simulink model "controller_lon2"  (R2017b)
settings: Solver=VariableStepAuto  StartTime=0.0  StopTime=10  RelTol=1e-3
values from neighbouring files (symbols this model uses):
  CSim_theta = 1    [controller_lon_design.m]
  KF_theta = 0.000000    (= 0)    [controller_lon_design.m]    (also in lon_gain20190526.mat = -0.572510862227)
  KI_theta = 0.3    [controller_lon_design.m]    (also in lon_gain20190526.mat = 0.842649674918)
  KP_q = 1.7    [controller_lon_design.m]    (also in lon_gain20190526.mat = 1.88196418813)
  KP_q2 = 0.3    [controller_lon_design.m]    (also in lon_gain20190526.mat = 0.215046441763)
  KP_theta = 1.2    [controller_lon_design.m]    (also in lon_gain20190526.mat = 0.644469729819)
undefined symbols (not defined in the file or in its folder): Actuators, Linmod
settings Model: Creator=zht  LastModifiedBy=zht

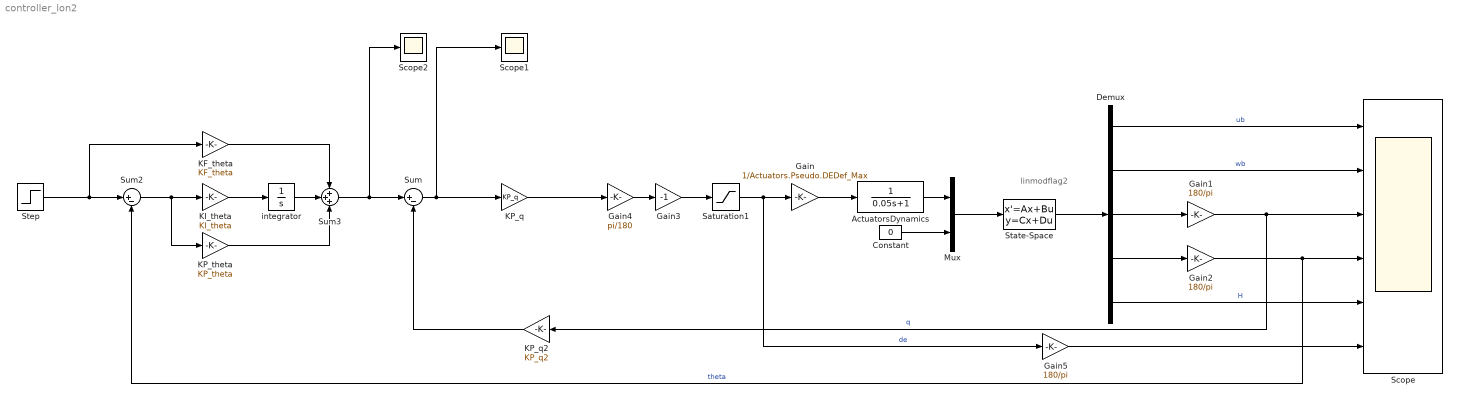
== system controller_lon2 ==
  note: linmodflag2
  ActuatorsDynamics : TransferFcn  Denominator=[0.05 1]
  Constant : Constant  Value=0
  Demux : Demux  Outputs=5
  Gain : Gain  Gain=1/Actuators.Pseudo.DEDef_Max
  Gain1 : Gain  Gain=180/pi
  Gain2 : Gain  Gain=180/pi
  Gain3 : Gain  Gain=-1
  Gain4 : Gain  Gain=pi/180
  Gain5 : Gain  Gain=180/pi
  KF_theta : Gain  Gain=KF_theta
  KI_theta : Gain  Gain=KI_theta
  KP_q : Gain  Gain=KP_q
  KP_q2 : Gain  Gain=KP_q2
  KP_theta : Gain  Gain=KP_theta
  Mux : Mux  Inputs=2
  Saturation1 : Saturate  UpperLimit=Actuators.Pseudo.DEDef_Max  LowerLimit=-Actuators.Pseudo.DEDef_Max
  Scope : Scope  NumInputPorts=6
  Scope1 : Scope
  Scope2 : Scope
  State-Space : StateSpace  A=Linmod.Lon_5.A  B=Linmod.Lon_5.B  C=Linmod.Lon_5.C  D=Linmod.Lon_5.D  InitialCondition=0  ContinuousStateAttributes={'ub','wb','q','theta','H'}
  Step : Step  Time=0  After=CSim_theta  SampleTime=0
  Sum : Sum  Inputs=|+-
  Sum2 : Sum  Inputs=|+-
  Sum3 : Sum  Inputs=+++
  integrator : Integrator
  wires:
  Mux/1 -> State-Space/1
  Constant/1 -> Mux/2
  State-Space/1 -> Demux/1
  Demux/2 -> Scope/2  "wb"
  Demux/3 -> Gain1/1
  Demux/4 -> Gain2/1
  Demux/5 -> Scope/5  "H"
  Demux/1 -> Scope/1  "ub"
  Gain1/1 -> KP_q2/1, Scope/3  "q"
  Gain2/1 -> Sum2/2, Scope/4  "theta"
  Gain/1 -> ActuatorsDynamics/1
  Sum/1 -> KP_q/1, Scope1/1
  Sum3/1 -> Scope2/1, Sum/1
  Sum2/1 -> KP_theta/1, KI_theta/1
  KP_q2/1 -> Sum/2
  Gain3/1 -> Saturation1/1
  ActuatorsDynamics/1 -> Mux/1
  Step/1 -> KF_theta/1, Sum2/1
  KP_q/1 -> Gain4/1
  integrator/1 -> Sum3/2
  KF_theta/1 -> Sum3/1
  KP_theta/1 -> Sum3/3
  KI_theta/1 -> integrator/1
  Saturation1/1 -> Gain5/1, Gain/1  "de"
  Gain4/1 -> Gain3/1
  Gain5/1 -> Scope/6
